simulink library "Valve"  (Simulink 8.2)
settings: Solver=ode45  StartTime=0.0  StopTime=10.0  RelTol=1e-3
undefined symbols (not defined in the file): DPConstant, DPLinear, DPQuadratic, ID, Pressure
libraries: carnot x1
settings Model: Creator=lena.frank  LastModifiedBy=drhf

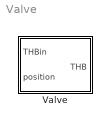
== system Valve ==
  Valve : Subsystem  mask(valve){pos_values=[0 0.1 1], dp_values=[1e6 1e6 1]}
      mask prompts: pos_values "position (vector with values 0..1)"; dp_values "QUA : quadratic pressure drop (vector)"
      mask help:
      | The block calculates the pressure drop at a valve. The characteristic is defined by a lookup table for QUA:
      | dp = QUA * mdot^2
      mask Help: web(fullfile(path_carnot('help'),'Valve.html'),'-helpbrowser')
      mask Display: plot(-15,0,115,100,[30,70,70,30,30],[60,40,60,40,60],[60,40],[80,80],[50,50],[50,80])

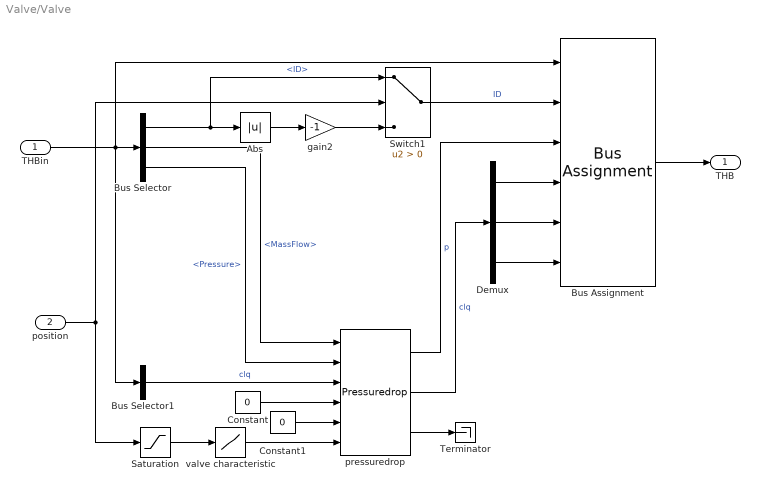
== system Valve/Valve ==
  THBin : Inport
  position : Inport  Port=2
  Abs : Abs
  Bus Assignment : BusAssignment  AssignedSignals=ID,Pressure,DPConstant,DPLinear,DPQuadratic
  Bus Selector : BusSelector  OutputSignals=ID,MassFlow,Pressure
  Bus Selector1 : BusSelector  OutputSignals=DPConstant,DPLinear,DPQuadratic  OutputAsBus=on
  Constant : Constant  Value=0
  Constant1 : Constant  Value=0
  Demux : Demux  Outputs=3
  Saturation : Saturate  UpperLimit=1  LowerLimit=0
  Switch1 : Switch  Criteria=u2 > Threshold  SaturateOnIntegerOverflow=on  InputSameDT=on
  Terminator : Terminator
  gain2 : Gain  Gain=-1  SaturateOnIntegerOverflow=on  OutDataTypeStr=Inherit: Same as input  ParamDataTypeStr=Inherit: Same as input
  pressuredrop : carnot/Basic/Pressure_Drop/Pressuredrop
  valve characteristic : Lookup  InputValues=pos_values  Table=dp_values  SaturateOnIntegerOverflow=on
  THB : Outport
  wires:
  gain2/1 -> Switch1/3
  Bus Selector/1 -> Switch1/1, Abs/1  "<ID>"
  position/1 -> Switch1/2, Saturation/1
  Bus Selector1/1 -> pressuredrop/3  "clq"
  pressuredrop/1 -> Bus Assignment/3  "p"
  Bus Selector/2 -> pressuredrop/1  "<MassFlow>"
  Saturation/1 -> valve characteristic/1
  Switch1/1 -> Bus Assignment/2  "ID"
  Abs/1 -> gain2/1
  Bus Selector/3 -> pressuredrop/2  "<Pressure>"
  pressuredrop/2 -> Demux/1  "clq"
  Constant/1 -> pressuredrop/4
  Constant1/1 -> pressuredrop/5
  valve characteristic/1 -> pressuredrop/6
  pressuredrop/3 -> Terminator/1
  THBin/1 -> Bus Selector/1, Bus Selector1/1, Bus Assignment/1
  Bus Assignment/1 -> THB/1
  Demux/1 -> Bus Assignment/4
  Demux/2 -> Bus Assignment/5
  Demux/3 -> Bus Assignment/6
